simulink model "PDController"  (R2021a)
settings: Solver=VariableStepAuto  StartTime=0.0  StopTime=10.0  RelTol=1e-3
libraries: robotlib x3
settings Model: Creator=nathanielgoldfarb  LastModifiedBy=nathanielgoldfarb

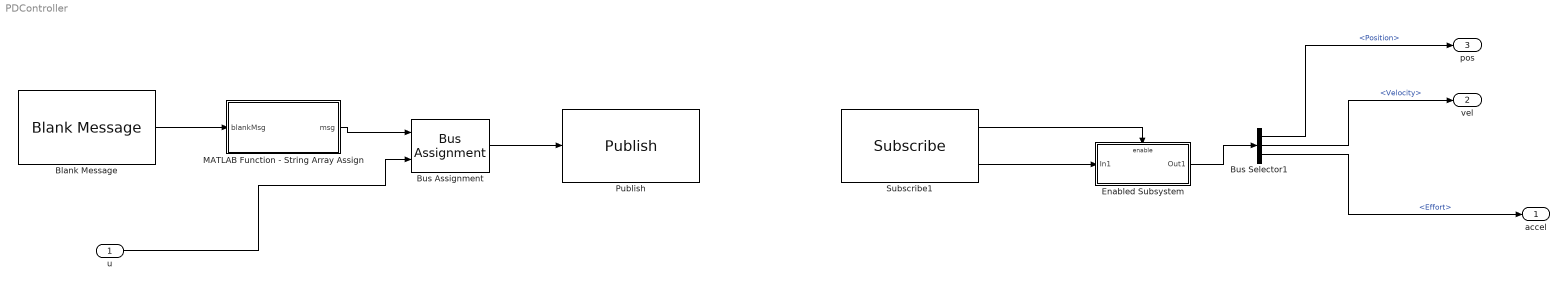
== system PDController ==
  u : Inport
  Blank Message : robotlib/Blank Message  messageClass=Message  entityType=sensor_msgs/JointState  messageType=sensor_msgs/JointState  SampleTime=inf  legacyBusStruct=off
  Bus Assignment : BusAssignment  AssignedSignals=Effort
  Bus Selector1 : BusSelector  OutputSignals=Position,Velocity,Effort
  Enabled Subsystem : Subsystem  TreatAsAtomicUnit=on
  MATLAB Function - String Array Assign : MATLAB Function  TreatAsAtomicUnit=on
  Publish : robotlib/Publish  topicSource=Select from ROS network  topic=/exo_simulink_torque  messageType=sensor_msgs/JointState  legacyBusStruct=off  messageQueueLength=1
  Subscribe1 : robotlib/Subscribe  topicSource=Select from ROS network  topic=/exo_jointstate  messageType=sensor_msgs/JointState  SampleTime=-1  legacyBusStruct=off  messageQueueLength=1
  accel : Outport
  vel : Outport  Port=2
  pos : Outport  Port=3
  wires:
  Blank Message/1 -> MATLAB Function - String Array Assign/1(blankMsg)
  Bus Selector1/1 -> pos/1  "<Position>"
  Enabled Subsystem/1(Out1) -> Bus Selector1/1
  MATLAB Function - String Array Assign/1(msg) -> Bus Assignment/1
  u/1 -> Bus Assignment/2
  Bus Assignment/1 -> Publish/1
  Subscribe1/1 -> Enabled Subsystem/Enable
  Bus Selector1/2 -> vel/1  "<Velocity>"
  Subscribe1/2 -> Enabled Subsystem/1(In1)
  Bus Selector1/3 -> accel/1  "<Effort>"

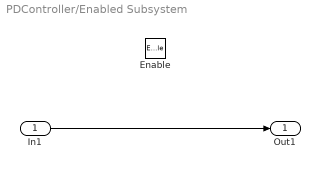
== system PDController/Enabled Subsystem ==
  In1 : Inport
  Enable : EnablePort
  Out1 : Outport
  wires:
  In1/1 -> Out1/1

== matlab function PDController/MATLAB Function - String Array Assign ==
  data: blankMsg input; msg output Bus: SL_Bus_PDController_sensor_msgs_JointState
function msg = stringArrayAssign(blankMsg)
% stringArrayAssign - Assign a string array in a ROS message
%
%  blankMsg (input): A bus for a 'sensor_msgs/JointState' message. This is 
%      used to initialize the output.
%  msg (output): A bus for a 'sensor_msgs/JointState' message message, with 
%      Name field set to a string array.
%
%   Copyright 2015 The MathWorks, Inc.

%#codegen

% Note: The datatype of 'msg' has been explicitly set to the appropriate 
% Simulink bus type ("SL_Bus_robotROSMessageUsageExample_sensor_msgs_JointState"). 
%
% If the model name is changed, the datatype needs to be changed as well:
%   1) Click "Edit Data" in the Editor toolstrip to open "Ports and Data Manager"
%   2) Select "msg". From the "Type" dropdown, select "--- Refresh data types ---"
%   3) Set datatype to "Bus: SL_Bus_<modelname>_sensor_msgs_JointState"

strArrayToAssign = {'LeftExoHip', 'LeftExoKnee', 'LeftExoAnkle', 'RightExoHip', 'RightExoKnee', 'RightExoAnkle', 'Crutches'};
msg = blankMsg;

% Set the number of strings in the string array.
% msg (sensor_msgs/JointState) includes the following fields
%           Name : array of std_msgs/String (string array)
%   Name_SL_Info : struct with fields CurrentLength, ReceivedLength
numStringsInArray = length(strArrayToAssign);
msg.Name_SL_Info.CurrentLength = uint32(numStringsInArray);
msg.Effort_SL_Info.CurrentLength = uint32(numStringsInArray);

% Set the individual strings in the array
for idx=1:numStringsInArray
    str = strArrayToAssign{idx};
    strLength = length(str);
    msg.Name(idx).Data(1:strLength) = uint8(str);
    msg.Name(idx).Data_SL_Info.CurrentLength = uint32(strLength);
end
